simulink model "first_simulink_m"  (R2021a)
settings: Solver=VariableStepAuto  StartTime=0.0  StopTime=10.0  RelTol=1e-3
settings Model: Creator=davidrico  LastModifiedBy=davidrico

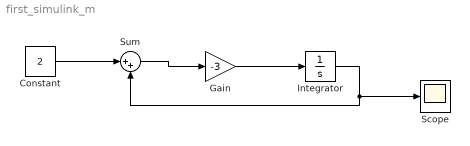
== system first_simulink_m ==
  Constant : Constant  Value=2
  Gain : Gain  Gain=-3
  Integrator : Integrator
  Scope : Scope
  Sum : Sum  Inputs=|++
  wires:
  Sum/1 -> Gain/1
  Gain/1 -> Integrator/1
  Integrator/1 -> Scope/1, Sum/2
  Constant/1 -> Sum/1
